simulink subsystem "subsys_calcul_Zk"  (R2021a)
settings: Solver=VariableStepAuto  StartTime=0.0  StopTime=10.0  RelTol=1e-3
settings Model: Creator=antho  LastModifiedBy=antho

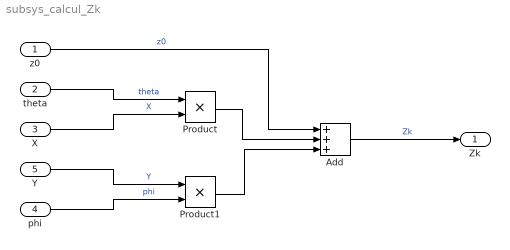
== system subsys_calcul_Zk ==
  z0 : Inport
  theta : Inport  Port=2
  X : Inport  Port=3
  phi : Inport  Port=4
  Y : Inport  Port=5
  Add : Sum  Inputs=+++
  Product : Product
  Product1 : Product
  Zk : Outport
  wires:
  Add/1 -> Zk/1  "Zk"
  Product1/1 -> Add/3
  Product/1 -> Add/2
  Y/1 -> Product1/1  "Y"
  z0/1 -> Add/1  "z0"
  X/1 -> Product/2  "X"
  theta/1 -> Product/1  "theta"
  phi/1 -> Product1/2  "phi"
